simulink model "initial_position"  (R2023a)
settings: Solver=VariableStepAuto  StartTime=0.0  StopTime=1  RelTol=1e-3
values from neighbouring files (symbols this model uses):
  m0 = 4    [position_control.m]    (also in satellite_model.m)
  mDot = 0.000102    [position_control.m]    (also in satellite_model.m)
  Ve = [Ve_x; 0; 0]    [position_control.m]    (also in satellite_model.m)
undefined symbols (not defined in the file or in its folder): juliandate
settings Model: Creator=shubi  LastModifiedBy=shubi

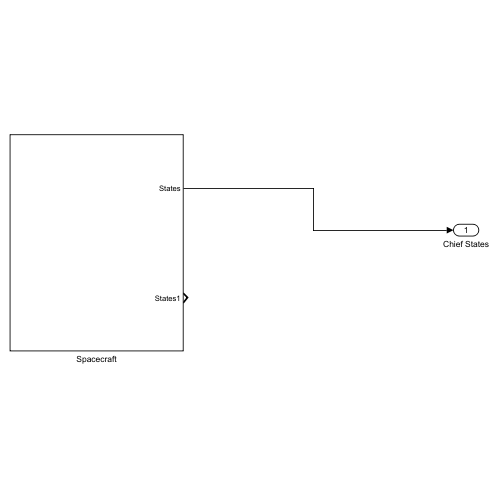
[thumbnail: Simulink's stored preview of the top-level diagram]
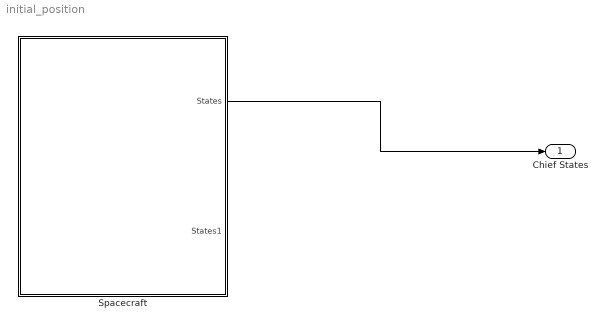
== system initial_position ==
  Spacecraft : Subsystem
  Chief States : Outport
  wires:
  Spacecraft/1(States) -> Chief States/1

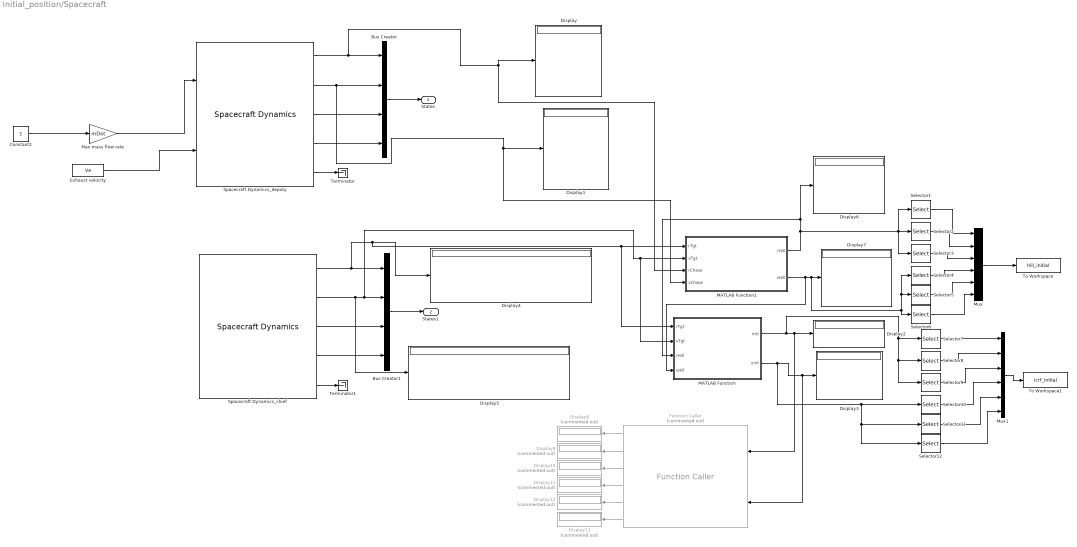
== system initial_position/Spacecraft ==
  Bus Creator : BusCreator  Inputs=4
  Bus Creator1 : BusCreator  Inputs=4
  Constant2 : Constant
  Display{,1..7} (8 alike) : Display
  Display{8..13} (6 alike) : Display  Commented=on
  Exhaust velocity : Constant  Value=Ve
  Function Caller : FunctionCaller  Commented=on  FunctionPrototype=[a,e,i,RAAN,omega,f] = rv2elem_si(rVec,vVec)  InputArgumentSpecifications=<Enter example>  OutputArgumentSpecifications=<Enter example>
  MATLAB Function : MATLAB Function  TreatAsAtomicUnit=on
  MATLAB Function1 : MATLAB Function  TreatAsAtomicUnit=on
  Max mass flow rate : Gain  Gain=mDot
  Mux : Mux  Inputs=6
  Mux1 : Mux  Inputs=6
  Selector{1,4,7,10} (4 alike) : Selector  InputPortWidth=3  IndexOptions=Index vector (dialog)  Indices=[1]  OutputSizes=1
  Selector{2,5,8,11} (4 alike) : Selector  InputPortWidth=3  IndexOptions=Index vector (dialog)  Indices=[2]  OutputSizes=1
  Selector{3,6,9,12} (4 alike) : Selector  InputPortWidth=3  IndexOptions=Index vector (dialog)  Indices=[3]  OutputSizes=1
  Spacecraft Dynamics_chief : SpacecraftDynamics  forcesIn=off  momentsIn=off  startDate=juliandate(2000, 1, 1, 12, 0, 0)  action=Error  mass=m0_C  emptyMass=m0-0.5  fullMass=m0  inertia=[600, 0, 0; 0, 500, 0; 0, 0, 550]  emptyInertia=[0.0058, 0, 0; 0, 0.0292, 0; 0, 0, 0.0292]  fullInertia=[0.0067, 0, 0; 0, 0.0333, 0; 0, 0, 0.0333]  useMassFlowRelativeVelocity=on  outputFuelStatus=off  semiMajorAxis=6878140  eccentricity=0  inclination=97.4065  raan=0  argPeriapsis=0  trueAnomaly=0  inertialPosition=[7229500.0, 4578700.0, -1432100.0]  attitude=[1, 0, 0,0]  attitudeRate=[-3, 2, 3]
  Spacecraft Dynamics_deputy : SpacecraftDynamics  forcesIn=off  momentsIn=off  startDate=juliandate(2000, 1, 1, 12, 0, 0)  action=Error  massType=Simple variable  mass=m0  emptyMass=m0-0.5  fullMass=m0  emptyInertia=[0.0058, 0, 0; 0, 0.0292, 0; 0, 0, 0.0292]  fullInertia=[0.0067, 0, 0; 0, 0.0333, 0; 0, 0, 0.0333]  useMassFlowRelativeVelocity=on  outputFuelStatus=off  semiMajorAxis=a  eccentricity=e  inclination=inc  raan=Omega  argPeriapsis=omega  trueAnomaly=f  inertialPosition=[7229600.0,4578800.0,-1432100.0]  inertialVelocity=[-3823.0, 6844.2, 2978.8]  attitude=[1, 0, 0,0]  attitudeRate=[-0.8, 0.4, 0.8]
  Terminator : Terminator
  Terminator1 : Terminator
  To Workspace : ToWorkspace  VariableName=hill_initial  SaveFormat=Timeseries  SampleTime=-1
      settings: Save2DSignal=2-D array (concatenate along first dimension)
  To Workspace1 : ToWorkspace  VariableName=icrf_initial  SaveFormat=Timeseries  SampleTime=-1
  States : Outport
  States1 : Outport  Port=2
  wires:
  Spacecraft Dynamics_deputy/3 -> Bus Creator/3
  Spacecraft Dynamics_deputy/4 -> Bus Creator/4
  Spacecraft Dynamics_deputy/5 -> Terminator/1
  Bus Creator/1 -> States/1
  Bus Creator1/1 -> States1/1
  Spacecraft Dynamics_chief/1 -> MATLAB Function/1(rTgt), MATLAB Function1/1(rTgt), Display4/1, Bus Creator1/1
  Spacecraft Dynamics_chief/4 -> Bus Creator1/4
  Spacecraft Dynamics_chief/2 -> Display5/1, MATLAB Function/2(vTgt), MATLAB Function1/2(vTgt), Bus Creator1/2
  Spacecraft Dynamics_chief/3 -> Bus Creator1/3
  Spacecraft Dynamics_chief/5 -> Terminator1/1
  MATLAB Function/2(vInt) -> Selector12/1, Selector11/1, Selector10/1, Function Caller/2, Display3/1
  Spacecraft Dynamics_deputy/2 -> MATLAB Function1/4(vChase), Display1/1, Bus Creator/2
  MATLAB Function1/1(rHill) -> Display6/1, MATLAB Function/3(rHill), Selector3/1, Selector2/1, Selector1/1
  MATLAB Function1/2(vHill) -> MATLAB Function/4(vHill), Selector4/1, Selector5/1, Selector6/1, Display7/1
  MATLAB Function/1(rInt) -> Selector9/1, Selector8/1, Selector7/1, Function Caller/1, Display2/1
  Function Caller/1 -> Display8/1
  Function Caller/2 -> Display9/1
  Function Caller/3 -> Display10/1
  Function Caller/4 -> Display11/1
  Function Caller/5 -> Display12/1
  Function Caller/6 -> Display13/1
  Constant2/1 -> Max mass flow rate/1
  Spacecraft Dynamics_deputy/1 -> MATLAB Function1/3(rChase), Display/1, Bus Creator/1
  Max mass flow rate/1 -> Spacecraft Dynamics_deputy/1
  Exhaust velocity/1 -> Spacecraft Dynamics_deputy/2
  Mux/1 -> To Workspace/1
  Mux1/1 -> To Workspace1/1
  Selector1/1 -> Mux/1
  Selector2/1 -> Mux/2
  Selector3/1 -> Mux/3
  Selector5/1 -> Mux/5
  Selector4/1 -> Mux/4
  Selector6/1 -> Mux/6
  Selector7/1 -> Mux1/1
  Selector12/1 -> Mux1/6
  Selector11/1 -> Mux1/5
  Selector10/1 -> Mux1/4
  Selector8/1 -> Mux1/2
  Selector9/1 -> Mux1/3

== matlab function initial_position/Spacecraft/MATLAB Function1 ==
  data: rTgt input; rHill output; vTgt input; rChase input; vChase input; vHill output
function [rHill,vHill] = ECI2Hill_Vectorized(rTgt,vTgt,rChase,vChase)
%% Purpose:
% Convert those position (ECI) and velocity (ECI) into Hill's reference
% frame using both the target and the chaser position/velocity data
%
%% Inputs:
%rTgt                       [3 x N]                 ECI Position vector of
%                                                   reference frame (km)
%
%vTgt                       [3 x N]                 ECI Velocity vector of
%                                                   reference frame (km/s)
%rChase                     [3 x N]
%
%vChase                     [3 x N]
%
%% Outputs:
%rHill                      [3 x N]                 Hill's relative
%                                                   position vector (km)
%
%vHill                      [3 x N]                 Hill's relative
%                                                   velocity vector (km/s)
% References:
% Vallado 2007.
% Programed by Darin C Koblick 11/30/2012

rTgt = rTgt *0.001;
vTgt = vTgt*0.001;
rChase = rChase*0.001;
vChase  =vChase*0.001;
%% Begin Code Sequence
%Declare Local Functions
matrixMultiply = @(x,y)permute(cat(2,sum(permute(x(1,:,:),[3 2 1]).*permute(y,[2 1]),2), ...
                                     sum(permute(x(2,:,:),[3 2 1]).*permute(y,[2 1]),2), ...
                                     sum(permute(x(3,:,:),[3 2 1]).*permute(y,[2 1]),2)),[2 1]);
rTgtMag = sqrt(sum(rTgt.^2,1));
rChaseMag = sqrt(sum(rChase.^2,1));
vTgtMag = sqrt(sum(vTgt.^2,1));
%Determine the RSW transformation matrix from the target frame of reference
RSW = ECI2RSW(rTgt,vTgt);
%Use RSW rotation matrix to convert rChase and vChase to RSW
r_Chase_RSW = matrixMultiply(RSW,rChase);
v_Chase_RSW = matrixMultiply(RSW,vChase);
%Find Rotation angles to go from target to interceptor
phi_chase = asin(r_Chase_RSW(3,:)./rChaseMag);
lambda_chase = atan2(r_Chase_RSW(2,:),r_Chase_RSW(1,:));
CPC = cos(phi_chase);     SPC = sin(phi_chase);
SLC = sin(lambda_chase);  CLC = cos(lambda_chase);
%Find Position component rotations
rHill = cat(1,rChaseMag-rTgtMag, ...
              lambda_chase.*rTgtMag, ...
              phi_chase.*rTgtMag);
%Find the rotation matrix RSW->SEZ of chaser
RSW_SEZ = zeros(3,3,size(rTgtMag,2));
RSW_SEZ(1,1,:) = SPC.*CLC;  RSW_SEZ(1,2,:) = SPC.*SLC;  RSW_SEZ(1,3,:) = -CPC;
RSW_SEZ(2,1,:) = -SLC;  RSW_SEZ(2,2,:) = CLC;
RSW_SEZ(3,1,:) = CPC.*CLC;  RSW_SEZ(3,2,:) = CPC.*SLC;  RSW_SEZ(3,3,:) = SPC;
%Find the velocity component of positions using the angular rates in SEZ frame
v_Chase_SEZ = matrixMultiply(RSW_SEZ,v_Chase_RSW);
vHill = cat(1,v_Chase_SEZ(3,:), ...
              rTgtMag.*(v_Chase_SEZ(2,:)./(rChaseMag.*CPC)-vTgtMag./rTgtMag), ...
              -rTgtMag.*v_Chase_SEZ(1,:)./rChaseMag);

rHill = rHill *1000;
vHill = vHill*1000;
end

function [T,rRSW,vRSW] = ECI2RSW(rECI,vECI)
%% Purpose:
%Convert ECI Coordinates to RSW Coordinates, also, return the
%transformation matrix T in which to take a given set of coordinates in ECI
%and convert them using the same RSW reference frame.
%
%% Inputs:
% rECI              [3 x N]                     ECI position Coordinates in
%                                               km
%
% vECI              [3 x N]                     ECI velocity Coordinates in
%                                               km/s
%
%% Outputs:
% T                 [3 x 3 x N]                 Transformation matrix
%                                               necessary to go from
%                                               rECI -> rRSW
%
% rRSW              [3 x N]                     RSW Position Coordinates
%                                               km
%
% vRSW              [3 x N]                     RSW Velocity Coordinates
%                                               km/s
%
%% References:
% Vallado pg. 173
% Vallado rv2rsw.m code dated 06/09/2002
%
%Programmed by: Darin C Koblick                 11/29/2012
%% Begin Code Sequence
if nargin == 0
    rECI =  repmat([6968.1363,1,2]',[1 10]);
    vECI =  repmat([3,7.90536615282099,4]',[1 10]);
    [T,rRSW,vRSW] = ECI2RSW(rECI,vECI);
    return;
end
%Declared Internal function set:
unitv = @(x)bsxfun(@rdivide,x,sqrt(sum(x.^2,1)));
matrixMultiply = @(x,y)permute(cat(2,sum(permute(x(1,:,:),[3 2 1]).*permute(y,[2 1]),2), ...
                                     sum(permute(x(2,:,:),[3 2 1]).*permute(y,[2 1]),2), ...
                                     sum(permute(x(3,:,:),[3 2 1]).*permute(y,[2 1]),2)),[2 1]);
%Find the Radial component of the RIC position vector
rvec = unitv(rECI);
%Find the cross-track component of the RIC position vector
wvec = unitv(cross(rECI,vECI));
%Find the along-track component of the RIC position vector
svec = unitv(cross(wvec,rvec));
%Create the transformation matrix from ECI to RSW
T = NaN(3,3,size(rECI,2));
T(1,1,:) = rvec(1,:); T(1,2,:) = rvec(2,:); T(1,3,:) = rvec(3,:);
T(2,1,:) = svec(1,:); T(2,2,:) = svec(2,:); T(2,3,:) = svec(3,:);
T(3,1,:) = wvec(1,:); T(3,2,:) = wvec(2,:); T(3,3,:) = wvec(3,:);
%Find the position and velocity vectors in the RSW reference frame!
rRSW = matrixMultiply(T,rECI);
vRSW = matrixMultiply(T,vECI);
end

== matlab function initial_position/Spacecraft/MATLAB Function ==
  data: rTgt input; rInt output; vTgt input; rHill input; vHill input; vInt output
function [rInt,vInt] = Hill2ECI_Vectorized(rTgt,vTgt,rHill,vHill)
%% Purpose:
% Convert those position (rHill) and velocity (vHill) values back into an
% ECI coordinate frame of reference using the reference satellite
% (rTgt,vTgt) position and velocity data.
%
%% Inputs:
%rTgt                       [3 x N]                 ECI Position vector of
%                                                   reference frame (km)
%
%vTgt                       [3 x N]                 ECI Velocity vector of
%                                                   reference frame (km/s)
%
%rHill                      [3 x N]                 Hill's relative
%                                                   position vector (km)
%
%vHill                      [3 x N]                 Hill's relative
%                                                   velocity vector (km/s)
%
%
%
%% Outputs:
%rInt                       [3 x N]
%
%vInt                       [3 x N]
%
%
% References:
% Vallado 2007.
% Programed by Darin C Koblick 11/30/2012

rTgt = rTgt *0.001;
vTgt = vTgt*0.001;
rHill = rHill*0.001;
vHill  =vHill*0.001;
%% Begin Code Sequence
%Declare Local Functions
rTgtMag = sqrt(sum(rTgt.^2,1));
vTgtMag = sqrt(sum(vTgt.^2,1));
matrixMultiply = @(x,y)permute(cat(2,sum(permute(x(1,:,:),[3 2 1]).*permute(y,[2 1]),2), ...
                                     sum(permute(x(2,:,:),[3 2 1]).*permute(y,[2 1]),2), ...
                                     sum(permute(x(3,:,:),[3 2 1]).*permute(y,[2 1]),2)),[2 1]);
%Find the RSW matrix from the target ECI positions
RSW = ECI2RSW(rTgt,vTgt); rIntMag = rTgtMag + rHill(1,:);
%Compute rotation angles to go from tgt to interceptor
lambda_int = rHill(2,:)./rTgtMag; phi_int = sin(rHill(3,:)./rTgtMag);
CLI = cos(lambda_int); SLI = sin(lambda_int); CPI = cos(phi_int); SPI = sin(phi_int);
%find rotation matrix to go from rsw to SEZ of inerceptor
RSW_SEZ = zeros(3,3,size(rTgt,2));
RSW_SEZ(1,1,:) = SPI.*CLI;  RSW_SEZ(1,2,:) = SPI.*SLI; RSW_SEZ(1,3,:) = -CPI;
RSW_SEZ(2,1,:) = -SLI;      RSW_SEZ(2,2,:) = CLI;      RSW_SEZ(3,1,:) = CPI.*CLI;
                            RSW_SEZ(3,2,:) = CPI.*SLI; RSW_SEZ(3,3,:) = SPI;
%Find velocity component positions by using angular rates in SEZ frame
vIntSEZ = cat(1,-rIntMag.*vHill(3,:)./rTgtMag, ...
                 rIntMag.*(vHill(2,:)./rTgtMag + vTgtMag./rTgtMag).*CPI, ...
                 vHill(1,:));
vInt = matrixMultiply(permute(RSW,[2 1 3]), ...
       matrixMultiply(permute(RSW_SEZ,[2 1 3]), ...
       vIntSEZ));
%Find the position components
rIntRSW = bsxfun(@times,rIntMag,cat(1,CPI.*CLI, ...
                                      CPI.*SLI, ...
                                      SPI));
rInt = matrixMultiply(permute(RSW,[2 1 3]),rIntRSW); 

rInt = rInt *1000;
vInt = vInt*1000;
end

function [T,rRSW,vRSW] = ECI2RSW(rECI,vECI)
%% Purpose:
%Convert ECI Coordinates to RSW Coordinates, also, return the
%transformation matrix T in which to take a given set of coordinates in ECI
%and convert them using the same RSW reference frame.
%
%% Inputs:
% rECI              [3 x N]                     ECI position Coordinates in
%                                               km
%
% vECI              [3 x N]                     ECI velocity Coordinates in
%                                               km/s
%
%% Outputs:
% T                 [3 x 3 x N]                 Transformation matrix
%                                               necessary to go from
%                                               rECI -> rRSW
%
% rRSW              [3 x N]                     RSW Position Coordinates
%                                               km
%
% vRSW              [3 x N]                     RSW Velocity Coordinates
%                                               km/s
%
%% References:
% Vallado pg. 173
% Vallado rv2rsw.m code dated 06/09/2002
%
%Programmed by: Darin C Koblick                 11/29/2012
%% Begin Code Sequence
if nargin == 0
    rECI =  repmat([6968.1363,1,2]',[1 10]);
    vECI =  repmat([3,7.90536615282099,4]',[1 10]);
    [T,rRSW,vRSW] = ECI2RSW(rECI,vECI);
    return;
end
%Declared Internal function set:
unitv = @(x)bsxfun(@rdivide,x,sqrt(sum(x.^2,1)));
matrixMultiply = @(x,y)permute(cat(2,sum(permute(x(1,:,:),[3 2 1]).*permute(y,[2 1]),2), ...
                                     sum(permute(x(2,:,:),[3 2 1]).*permute(y,[2 1]),2), ...
                                     sum(permute(x(3,:,:),[3 2 1]).*permute(y,[2 1]),2)),[2 1]);
%Find the Radial component of the RIC position vector
rvec = unitv(rECI);
%Find the cross-track component of the RIC position vector
wvec = unitv(cross(rECI,vECI));
%Find the along-track component of the RIC position vector
svec = unitv(cross(wvec,rvec));
%Create the transformation matrix from ECI to RSW
T = NaN(3,3,size(rECI,2));
T(1,1,:) = rvec(1,:); T(1,2,:) = rvec(2,:); T(1,3,:) = rvec(3,:);
T(2,1,:) = svec(1,:); T(2,2,:) = svec(2,:); T(2,3,:) = svec(3,:);
T(3,1,:) = wvec(1,:); T(3,2,:) = wvec(2,:); T(3,3,:) = wvec(3,:);
%Find the position and velocity vectors in the RSW reference frame!
rRSW = matrixMultiply(T,rECI);
vRSW = matrixMultiply(T,vECI);
end
